simulink model "dcsimul"  (R2021b)
settings: Solver=ode4  StartTime=0.0  StopTime=30  FixedStep=ts  RelTol=1e-3
values from neighbouring files (symbols this model uses):
  A = [ -R/L -K_hat/L 0 ... (first row only)    [dc_sim_inpgps.m]    (also in in_gps_est.m = [ -R_hat/L_hat -K/L_hat 0; untitled.m = [ -R_hat/L_hat -K_hat/L_hat 0)
  a0 = param(3)    [in_gps_est.m]
  a1 = param(2)    [in_gps_est.m]
  a2 = param(1)    [in_gps_est.m]
  B = [ 1/L; 0 ; 0]    [dc_sim_inpgps.m]    (also in in_gps_est.m = [ 1/L_hat; 0 ; 0]; untitled.m = [ 1/L_hat; 0 ; 0])
  C = eye(3)    [dc_sim_inpgps.m]    (also in in_gps_est.m; untitled.m)
  D = [0;0;0;]    [dc_sim_inpgps.m]    (also in in_gps_est.m; untitled.m)
  Kas = 1/Kps    [in_gps_est.m]
  ts = 0.0005    [dc_motor_ingps.m]    (also in dc_sim_inpgps.m; in_gps_est.m; untitled.m)
undefined symbols (not defined in the file or in its folder): A1, B1, C1, D1
libraries: simulink x1
settings Model: Creator=JongBeom  LastModifiedBy=JongBeom
settings DataIOCC: ReturnWorkspaceOutputs=off

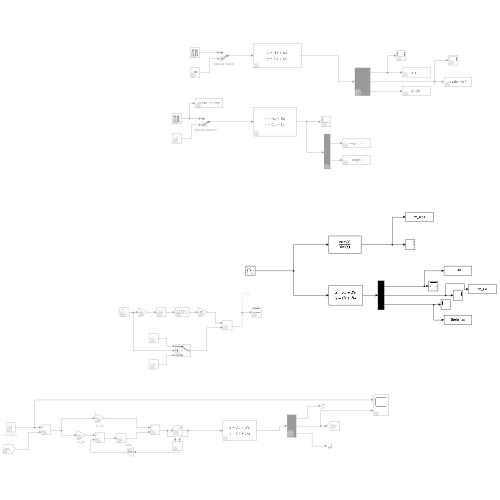
[thumbnail: Simulink's stored preview of the top-level diagram]
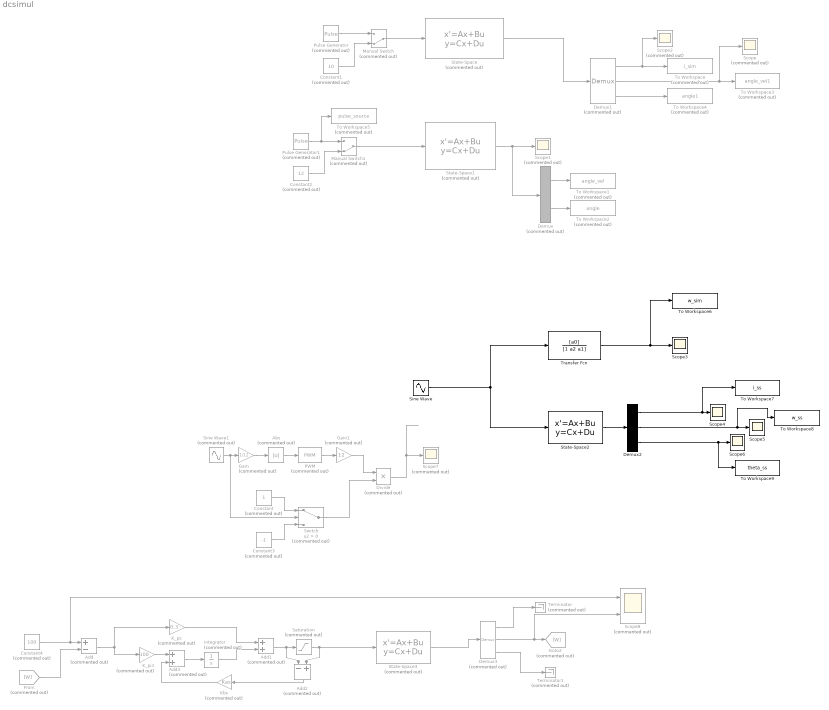
== system dcsimul ==
  Abs : Abs  Commented=on
  Add : Sum  Commented=on  Inputs=+-
  Add1 : Sum  Commented=on
  Add2 : Sum  Commented=on  Inputs=-+
  Add3 : Sum  Commented=on
  Constant : Constant  Commented=on
  Constant1 : Constant  Commented=on  Value=10
  Constant2 : Constant  Commented=on  Value=12
  Constant3 : Constant  Commented=on  Value=-1
  Constant4 : Constant  Commented=on  Value=100
  Demux : Demux  Commented=on  Outputs=2
  Demux1 : Demux  Commented=on  Outputs=3
  Demux2 : Demux  Outputs=3
  Demux3 : Demux  Commented=on  Outputs=3
  Divide : Product  Commented=on  Inputs=**
  From : From  Commented=on  GotoTag=W
  Gain : Gain  Commented=on  Gain=1/12
  Gain1 : Gain  Commented=on  Gain=12
  Goto2 : Goto  Commented=on  GotoTag=W
  Integrator : Integrator  Commented=on
  K_pi1 : Gain  Commented=on  Gain=100
  K_ps : Gain  Commented=on  Gain=0.3
  Kbs : Gain  Commented=on  Gain=Kas
  Manual Switch : ManualSwitch  Commented=on  CurrentSetting=0
  Manual Switch1 : ManualSwitch  Commented=on  CurrentSetting=0
  PWM : simulink/Discontinuities/PWM  Commented=on  DisableCoverage=on  Period=1/10000  DisallowZeroDutyCycle=off  RunAtFixedTimeIntervals=off  SampleTime=ts
  Pulse Generator : DiscretePulseGenerator  Commented=on  PulseType=Time based  Amplitude=12  Period=0.02  PulseWidth=50
  Pulse Generator1 : DiscretePulseGenerator  Commented=on  PulseType=Time based  Amplitude=12  Period=0.02  PulseWidth=50
  Saturation : Saturate  Commented=on  UpperLimit=12  LowerLimit=-12
  Scope{,1..2,7} (4 alike) : Scope  Commented=on
  Scope{3..6} (4 alike) : Scope
  Scope8 : Scope  Commented=on  NumInputPorts=2
  Sine Wave : Sin  Amplitude=10  Frequency=2  SampleTime=0
  Sine Wave1 : Sin  Commented=on  Amplitude=10  SampleTime=0
  State-Space : StateSpace  Commented=on  A=A  B=B  C=C  D=D  InitialCondition=0
  State-Space1 : StateSpace  Commented=on  A=A1  B=B1  C=C1  D=D1  InitialCondition=0
  State-Space2 : StateSpace  A=A  B=B  C=C  D=D  InitialCondition=0
  State-Space3 : StateSpace  Commented=on  A=A  B=B  C=C  D=D  InitialCondition=0
  Switch : Switch  Commented=on  Criteria=u2 > Threshold
  Terminator : Terminator  Commented=on
  Terminator1 : Terminator  Commented=on
  To Workspace : ToWorkspace  Commented=on  VariableName=i_sim  SampleTime=-1
  To Workspace1 : ToWorkspace  Commented=on  VariableName=angle_vel  SampleTime=-1
  To Workspace2 : ToWorkspace  Commented=on  VariableName=angle  SampleTime=-1
  To Workspace3 : ToWorkspace  Commented=on  VariableName=angle_vel1  SampleTime=-1
  To Workspace4 : ToWorkspace  Commented=on  VariableName=angle1  SampleTime=-1
  To Workspace5 : ToWorkspace  Commented=on  VariableName=pulse_source  SampleTime=-1
  To Workspace6 : ToWorkspace  VariableName=w_sim  SampleTime=-1
  To Workspace7 : ToWorkspace  VariableName=i_ss  SampleTime=-1
  To Workspace8 : ToWorkspace  VariableName=w_ss  SampleTime=-1
  To Workspace9 : ToWorkspace  VariableName=theta_ss  SampleTime=-1
  Transfer Fcn : TransferFcn  Numerator=[a0]  Denominator=[1 a2 a1]
  wires:
  Manual Switch1/1 -> State-Space1/1
  State-Space/1 -> Demux1/1
  State-Space1/1 -> Demux/1, Scope1/1
  Demux/1 -> To Workspace1/1
  Demux/2 -> To Workspace2/1
  Pulse Generator/1 -> Manual Switch/1
  Constant1/1 -> Manual Switch/2
  Manual Switch/1 -> State-Space/1
  Demux1/3 -> To Workspace4/1
  Demux1/2 -> Scope/1, To Workspace3/1
  Pulse Generator1/1 -> To Workspace5/1, Manual Switch1/1
  Constant2/1 -> Manual Switch1/2
  Demux1/1 -> Scope2/1, To Workspace/1
  Transfer Fcn/1 -> To Workspace6/1, Scope3/1
  State-Space2/1 -> Demux2/1
  Demux2/2 -> To Workspace8/1, Scope5/1
  Demux2/3 -> To Workspace9/1, Scope6/1
  Sine Wave1/1 -> Switch/2, Gain/1
  Gain/1 -> Abs/1
  Sine Wave/1 -> Transfer Fcn/1, State-Space2/1
  PWM/1 -> Gain1/1
  Abs/1 -> PWM/1
  Gain1/1 -> Divide/1
  Divide/1 -> Scope7/1
  Constant/1 -> Switch/1
  Constant3/1 -> Switch/3
  Switch/1 -> Divide/2
  Demux2/1 -> To Workspace7/1, Scope4/1
  Saturation/1 -> State-Space3/1, Add2/2
  Add3/1 -> Integrator/1
  K_pi1/1 -> Add3/1
  Kbs/1 -> Add3/2
  K_ps/1 -> Add1/1
  Add2/1 -> Kbs/1
  Integrator/1 -> Add1/2
  Add1/1 -> Add2/1, Saturation/1
  Add/1 -> K_ps/1, K_pi1/1
  State-Space3/1 -> Demux3/1
  Demux3/1 -> Terminator/1
  Demux3/2 -> Scope8/2, Goto2/1
  Demux3/3 -> Terminator1/1
  From/1 -> Add/2
  Constant4/1 -> Scope8/1, Add/1
